simulink model "Encoder_reader_simulink"  (R2025b)
settings: Solver=FixedStepAuto  StartTime=0.0  StopTime=inf  FixedStep=0.01  RelTol=1e-3  EnableMultiTasking=on
libraries: stm32g4xxblockslib x4, stm32f4xxblockslib x2
settings Model: STM32="{\"EncoderBlockForG4\":[{\"ID\":\"untitled:1\"},{\"ID\":\"Lab3_Encoder:1\"},{\"ID\":\"Encoder_reader_simulink:1\"},{\"ID\":\"Encoder_reader_simulink:52\"},{\"ID\":\"Encoder_reader_simulink:53\"},{\"ID\":\"Encoder_reader_simulink:109\"}],\"DigitalPortRead\":[{\"ID\":\"Encoder_reader_simulink:40\"},{\"ID\":\"Encoder_reader_simulink:41\"}]}"  SimulationMode=external  Creator=User  LastModifiedBy=gongk
settings OptimizationCC: DefaultParameterBehavior=Inlined  EnhancedBackFolding=on  PassReuseOutputArgsAs=Individual arguments  ZeroExternalMemoryAtStartup=off  ZeroInternalMemoryAtStartup=off  MaxStackSize=512  OptimizeBlockOrder=speed  DifferentSizesBufferReuse=on  OptimizationCustomize=off  EfficientTunableParamExpr=on
settings DebuggingCC: ParameterTunabilityLossMsg=error
settings HardwareCC: ProdBitPerPointer=32.0  ProdBitPerSizeT=32.0  ProdBitPerPtrDiffT=32.0  ProdLargestAtomicInteger=Long  ProdLargestAtomicFloat=Double  ProdWordSize=32.0  ProdLongLongMode=on  ProdHWDeviceType=ARM Compatible->ARM Cortex-M
settings SFSimCC: MATLABDynamicMemAlloc=off
settings RTWCC: SystemTargetFile=ert.tlc  HardwareBoard=STM32G4xx Based  TemplateMakefile=ert_default_tmf  Toolchain=GNU Tools for ARM Embedded Processors  Description=Embedded Coder
settings CodeAppCC: ForceParamTrailComments=on  IgnoreCustomStorageClasses=off  OperatorAnnotations=on  SimulinkDataObjDesc=on  SFDataObjDesc=on  InsertBlockDesc=on
settings ERTTargetCC: ExtModeTransport=3.0  ExtModeStaticAlloc=on  ExtModeStaticAllocSize=2048.0  ExtModeMexFile=ext_xcp  ExtModeIntrfLevel=Level2 - Open  TargetLangStandard=C99 (ISO)  CodeReplacementLibrary=ARM Cortex-M  SupportContinuousTime=on

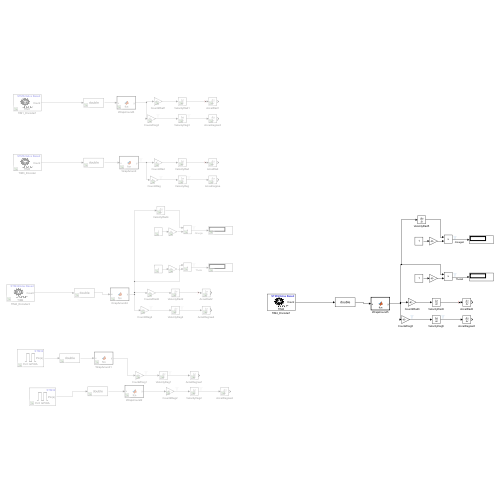
[thumbnail: Simulink's stored preview of the top-level diagram]
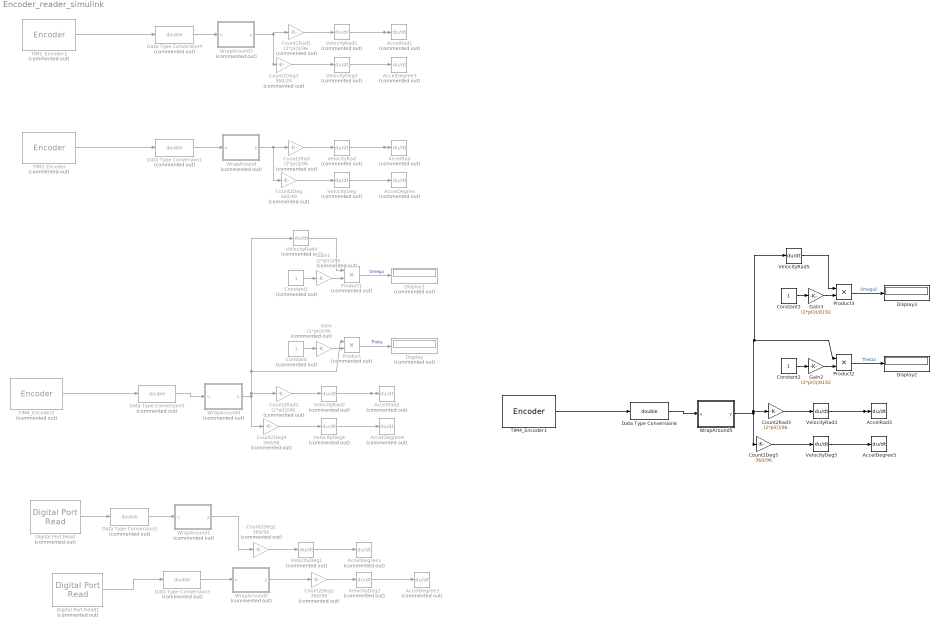
== system Encoder_reader_simulink ==
  AccelDegree{,1..4} (5 alike) : Derivative  Commented=on
  AccelDegree5 : Derivative
  AccelRad : Derivative  Commented=on
  AccelRad1 : Derivative  Commented=on
  AccelRad2 : Derivative  Commented=on
  AccelRad3 : Derivative
  Constant : Constant  Commented=on
  Constant1 : Constant  Commented=on
  Constant2 : Constant
  Constant3 : Constant
  Count2Deg : Gain  Commented=on  Gain=360/48
  Count2Deg1 : Gain  Commented=on  Gain=360/96
  Count2Deg2 : Gain  Commented=on  Gain=360/96
  Count2Deg3 : Gain  Commented=on  Gain=360/24
  Count2Deg4 : Gain  Commented=on  Gain=360/96
  Count2Deg5 : Gain  Gain=360/96
  Count2Rad : Gain  Commented=on  Gain=(2*pi())/96
  Count2Rad1 : Gain  Commented=on  Gain=(2*pi())/96
  Count2Rad2 : Gain  Commented=on  Gain=(2*pi())/96
  Count2Rad3 : Gain  Gain=(2*pi())/96
  Data Type Conversion{1..5} (5 alike) : DataTypeConversion  Commented=on  OutDataTypeStr=double  SaturateOnIntegerOverflow=off  RndMeth=Floor
  Data Type Conversion6 : DataTypeConversion  OutDataTypeStr=double  SaturateOnIntegerOverflow=off  RndMeth=Floor
  Digital Port Read : stm32f4xxblockslib/Digital Port Read  Commented=on  PortName=GPIOA  PinNumber=[4]  ReadOperation=on  IOAsArray=on  SampleTime=-1  EnableSimPort=off  hoistedMaskSrc=ECSoC/ECSimCodegen/Digital Port Read
  Digital Port Read1 : stm32f4xxblockslib/Digital Port Read  Commented=on  PortName=GPIOA  PinNumber=[6]  ReadOperation=on  IOAsArray=on  SampleTime=-1  EnableSimPort=off  hoistedMaskSrc=ECSoC/ECSimCodegen/Digital Port Read
  Display : Display  Commented=on
  Display1 : Display  Commented=on
  Display2 : Display
  Display3 : Display
  Gain : Gain  Commented=on  Gain=(2*pi())/96
  Gain1 : Gain  Commented=on  Gain=(2*pi())/96
  Gain2 : Gain  Gain=(2*pi())/8192
  Gain3 : Gain  Gain=(2*pi())/8192
  Product : Product  Commented=on
  Product1 : Product  Commented=on
  Product2 : Product
  Product3 : Product
  TIM1_Encoder1 : stm32g4xxblockslib/Encoder  Commented=on  TimerModule=TIM1  EnableResetInput=off  OutputCountAfterFirstIndex=off  OutputValidIndex=off  OutputDirection=off  OutputStatus=off  SampleTime=-1
  TIM3_Encoder : stm32g4xxblockslib/Encoder  Commented=on  TimerModule=TIM3  EnableResetInput=off  OutputCountAfterFirstIndex=off  OutputValidIndex=off  OutputDirection=off  OutputStatus=off  SampleTime=-1
  TIM4_Encoder1 : stm32g4xxblockslib/Encoder  TimerModule=TIM4  EnableResetInput=off  OutputCountAfterFirstIndex=off  OutputValidIndex=off  OutputDirection=off  OutputStatus=off  SampleTime=-1
  TIM4_Encoder2 : stm32g4xxblockslib/Encoder  Commented=on  TimerModule=TIM4  EnableResetInput=off  OutputCountAfterFirstIndex=off  OutputValidIndex=off  OutputDirection=off  OutputStatus=off  SampleTime=-1
  VelocityDeg{,1..4} (5 alike) : Derivative  Commented=on
  VelocityDeg5 : Derivative
  VelocityRad{,1..2,4} (4 alike) : Derivative  Commented=on
  VelocityRad3 : Derivative
  VelocityRad5 : Derivative
  WrapAround : MATLAB Function  Commented=on  TreatAsAtomicUnit=on
  WrapAround1 : MATLAB Function  Commented=on  TreatAsAtomicUnit=on
  WrapAround2 : MATLAB Function  Commented=on  TreatAsAtomicUnit=on
  WrapAround3 : MATLAB Function  Commented=on  TreatAsAtomicUnit=on
  WrapAround4 : MATLAB Function  Commented=on  TreatAsAtomicUnit=on
  WrapAround5 : MATLAB Function  TreatAsAtomicUnit=on
  wires:
  TIM3_Encoder/1 -> Data Type Conversion1/1
  Data Type Conversion1/1 -> WrapAround/1(u)
  WrapAround/1(y) -> Count2Deg/1, Count2Rad/1
  Count2Rad/1 -> VelocityRad/1
  Count2Deg/1 -> VelocityDeg/1
  VelocityDeg/1 -> AccelDegree/1
  VelocityRad/1 -> AccelRad/1
  VelocityDeg1/1 -> AccelDegree1/1
  Count2Deg1/1 -> VelocityDeg1/1
  WrapAround1/1(y) -> Count2Deg1/1
  Digital Port Read/1 -> Data Type Conversion2/1
  Data Type Conversion2/1 -> WrapAround1/1(u)
  Digital Port Read1/1 -> Data Type Conversion3/1
  Data Type Conversion3/1 -> WrapAround2/1(u)
  WrapAround2/1(y) -> Count2Deg2/1
  VelocityDeg2/1 -> AccelDegree2/1
  Count2Deg2/1 -> VelocityDeg2/1
  VelocityDeg3/1 -> AccelDegree3/1
  VelocityRad1/1 -> AccelRad1/1
  Count2Deg3/1 -> VelocityDeg3/1
  WrapAround3/1(y) -> Count2Rad1/1, Count2Deg3/1
  Count2Rad1/1 -> VelocityRad1/1
  Data Type Conversion4/1 -> WrapAround3/1(u)
  VelocityDeg4/1 -> AccelDegree4/1
  VelocityRad2/1 -> AccelRad2/1
  Count2Deg4/1 -> VelocityDeg4/1
  WrapAround4/1(y) -> VelocityRad4/1, Product/1, Count2Rad2/1, Count2Deg4/1
  Count2Rad2/1 -> VelocityRad2/1
  Data Type Conversion5/1 -> WrapAround4/1(u)
  TIM4_Encoder2/1 -> Data Type Conversion5/1
  TIM1_Encoder1/1 -> Data Type Conversion4/1
  Constant/1 -> Gain/1
  Gain/1 -> Product/2
  Product/1 -> Display/1  "Theta"
  VelocityRad4/1 -> Product1/1
  Gain1/1 -> Product1/2
  Product1/1 -> Display1/1  "Omega"
  Constant1/1 -> Gain1/1
  Constant3/1 -> Gain3/1
  Gain3/1 -> Product3/2
  Product3/1 -> Display3/1  "Omega2"
  VelocityRad5/1 -> Product3/1
  Gain2/1 -> Product2/2
  Product2/1 -> Display2/1  "Theta2"
  Constant2/1 -> Gain2/1
  Count2Rad3/1 -> VelocityRad3/1
  VelocityDeg5/1 -> AccelDegree5/1
  Count2Deg5/1 -> VelocityDeg5/1
  Data Type Conversion6/1 -> WrapAround5/1(u)
  TIM4_Encoder1/1 -> Data Type Conversion6/1
  VelocityRad3/1 -> AccelRad3/1
  WrapAround5/1(y) -> VelocityRad5/1, Product2/1, Count2Rad3/1, Count2Deg5/1

== matlab function Encoder_reader_simulink/WrapAround ==
  data: u input; y output
function y = fcn(u)
% fcn(u) - ฟังก์ชันสำหรับจัดการ Encoder Wrap-Around
% u: คือ Input (ค่าดิบจาก TIM3 ที่เป็น double)
% y: คือ Output (ค่าตำแหน่งสะสมที่ต่อเนื่อง)

%#codegen

% --- 1. กำหนดค่าคงที่ ---
% ค่า Counter Period (ARR) ที่ตั้งใน IOC คือ 61439
% ดังนั้น จำนวนนับทั้งหมด (States) คือ 61439 + 1 = 61440
persistent PERIOD;
persistent HALF_PERIOD;

% --- 2. สร้างตัวแปร "จำ" ค่า (Persistent Variables) ---
% persistent คือตัวแปรที่ "จำ" ค่าของตัวเองไว้ได้ แม้ฟังก์ชันจะรันจบไปแล้ว
persistent last_raw_count;    % เก็บค่าดิบจาก TIM3 ครั้งล่าสุด
persistent accumulated_count; % เก็บค่าตำแหน่งสะสม (Output)

% --- 3. การรันครั้งแรก (Initialization) ---
% isempty() จะเป็นจริงแค่ครั้งแรกที่ Simulink เริ่มรัน
if isempty(PERIOD)
    PERIOD        = 61440.0; % 61439 + 1 (ใช้ .0 เพื่อให้เป็น double)
    HALF_PERIOD   = PERIOD / 2.0; % 30720.0 
end

if isempty(last_raw_count)
    % ถ้าเป็นครั้งแรก ให้ตั้งค่าเริ่มต้น
    last_raw_count    = u;
    accumulated_count = 0.0;
else
    % --- 4. การรันครั้งถัดๆ ไป (คำนวณหาค่าต่าง) ---
    
    % หาผลต่างดิบ (Raw Delta)
    delta = u - last_raw_count;
    
    % --- 5. ตรวจจับการวนกลับ (Wrap-Around Detection) ---
    
    if delta < -HALF_PERIOD
        % เกิด Overflow (เช่น จาก 61439 -> 0, delta จะประมาณ -61439)
        % นี่คือการหมุนไปข้างหน้า (+1)
        delta = delta + PERIOD; % แก้ไข: -61439 + 61440 = +1
        
    elseif delta > HALF_PERIOD
        % เกิด Underflow (เช่น จาก 0 -> 61439, delta จะประมาณ +61439)
        % นี่คือการหมุนย้อนกลับ (-1)
        delta = delta - PERIOD; % แก้ไข: +61439 - 61440 = -1
    
    % else: (ถ้า delta อยู่ในช่วง +/- 30720)
        % ไม่มีการวนกลับ, 'delta' ถูกต้องแล้ว
    end
    
    % --- 6. อัปเดตค่าสะสม และค่าล่าสุด ---
    
    % บวกค่า delta ที่แก้ไขแล้ว เข้าไปในค่าสะสม
    accumulated_count = accumulated_count + delta;


    
    % "จำ" ค่าดิบครั้งนี้ไว้ เพื่อใช้ในรอบถัดไป
    last_raw_count = u;
end

% --- 7. ส่งค่า Output ---
y = accumulated_count;

end

== matlab function Encoder_reader_simulink/WrapAround2 ==
  data: u input; y output
function y = fcn(u)
% fcn(u) - ฟังก์ชันสำหรับจัดการ Encoder Wrap-Around
% u: คือ Input (ค่าดิบจาก TIM3 ที่เป็น double)
% y: คือ Output (ค่าตำแหน่งสะสมที่ต่อเนื่อง)

%#codegen

% --- 1. กำหนดค่าคงที่ ---
% ค่า Counter Period (ARR) ที่ตั้งใน IOC คือ 61439
% ดังนั้น จำนวนนับทั้งหมด (States) คือ 61439 + 1 = 61440
persistent PERIOD;
persistent HALF_PERIOD;

% --- 2. สร้างตัวแปร "จำ" ค่า (Persistent Variables) ---
% persistent คือตัวแปรที่ "จำ" ค่าของตัวเองไว้ได้ แม้ฟังก์ชันจะรันจบไปแล้ว
persistent last_raw_count;    % เก็บค่าดิบจาก TIM3 ครั้งล่าสุด
persistent accumulated_count; % เก็บค่าตำแหน่งสะสม (Output)

% --- 3. การรันครั้งแรก (Initialization) ---
% isempty() จะเป็นจริงแค่ครั้งแรกที่ Simulink เริ่มรัน
if isempty(PERIOD)
    PERIOD        = 1024.0; % 61439 + 1 (ใช้ .0 เพื่อให้เป็น double)
    HALF_PERIOD   = PERIOD / 2.0; % 30720.0 
end

if isempty(last_raw_count)
    % ถ้าเป็นครั้งแรก ให้ตั้งค่าเริ่มต้น
    last_raw_count    = u;
    accumulated_count = u;
else
    % --- 4. การรันครั้งถัดๆ ไป (คำนวณหาค่าต่าง) ---
    
    % หาผลต่างดิบ (Raw Delta)
    delta = u - last_raw_count;
    
    % --- 5. ตรวจจับการวนกลับ (Wrap-Around Detection) ---
    
    if delta < -HALF_PERIOD
        % เกิด Overflow (เช่น จาก 61439 -> 0, delta จะประมาณ -61439)
        % นี่คือการหมุนไปข้างหน้า (+1)
        delta = delta + PERIOD; % แก้ไข: -61439 + 61440 = +1
        
    elseif delta > HALF_PERIOD
        % เกิด Underflow (เช่น จาก 0 -> 61439, delta จะประมาณ +61439)
        % นี่คือการหมุนย้อนกลับ (-1)
        delta = delta - PERIOD; % แก้ไข: +61439 - 61440 = -1
    
    % else: (ถ้า delta อยู่ในช่วง +/- 30720)
        % ไม่มีการวนกลับ, 'delta' ถูกต้องแล้ว
    end
    
    % --- 6. อัปเดตค่าสะสม และค่าล่าสุด ---
    
    % บวกค่า delta ที่แก้ไขแล้ว เข้าไปในค่าสะสม
    accumulated_count = accumulated_count + delta;
    
    % "จำ" ค่าดิบครั้งนี้ไว้ เพื่อใช้ในรอบถัดไป
    last_raw_count = u;
end

% --- 7. ส่งค่า Output ---
y = accumulated_count;

end

== matlab function Encoder_reader_simulink/WrapAround3 ==
  data: u input; y output
function y = fcn(u)
% fcn(u) - ฟังก์ชันสำหรับจัดการ Encoder Wrap-Around
% u: คือ Input (ค่าดิบจาก TIM3 ที่เป็น double)
% y: คือ Output (ค่าตำแหน่งสะสมที่ต่อเนื่อง)

%#codegen

% --- 1. กำหนดค่าคงที่ ---
% ค่า Counter Period (ARR) ที่ตั้งใน IOC คือ 61439
% ดังนั้น จำนวนนับทั้งหมด (States) คือ 61439 + 1 = 61440
persistent PERIOD;
persistent HALF_PERIOD;

% --- 2. สร้างตัวแปร "จำ" ค่า (Persistent Variables) ---
% persistent คือตัวแปรที่ "จำ" ค่าของตัวเองไว้ได้ แม้ฟังก์ชันจะรันจบไปแล้ว
persistent last_raw_count;    % เก็บค่าดิบจาก TIM3 ครั้งล่าสุด
persistent accumulated_count; % เก็บค่าตำแหน่งสะสม (Output)

% --- 3. การรันครั้งแรก (Initialization) ---
% isempty() จะเป็นจริงแค่ครั้งแรกที่ Simulink เริ่มรัน
if isempty(PERIOD)
    PERIOD        = 61440.0; % 61439 + 1 (ใช้ .0 เพื่อให้เป็น double)
    HALF_PERIOD   = PERIOD / 2.0; % 30720.0 
end

if isempty(last_raw_count)
    % ถ้าเป็นครั้งแรก ให้ตั้งค่าเริ่มต้น
    last_raw_count    = u;
    accumulated_count = 0.0;
else
    % --- 4. การรันครั้งถัดๆ ไป (คำนวณหาค่าต่าง) ---
    
    % หาผลต่างดิบ (Raw Delta)
    delta = u - last_raw_count;
    
    % --- 5. ตรวจจับการวนกลับ (Wrap-Around Detection) ---
    
    if delta < -HALF_PERIOD
        % เกิด Overflow (เช่น จาก 61439 -> 0, delta จะประมาณ -61439)
        % นี่คือการหมุนไปข้างหน้า (+1)
        delta = delta + PERIOD; % แก้ไข: -61439 + 61440 = +1
        
    elseif delta > HALF_PERIOD
        % เกิด Underflow (เช่น จาก 0 -> 61439, delta จะประมาณ +61439)
        % นี่คือการหมุนย้อนกลับ (-1)
        delta = delta - PERIOD; % แก้ไข: +61439 - 61440 = -1
    
    % else: (ถ้า delta อยู่ในช่วง +/- 30720)
        % ไม่มีการวนกลับ, 'delta' ถูกต้องแล้ว
    end
    
    % --- 6. อัปเดตค่าสะสม และค่าล่าสุด ---
    
    % บวกค่า delta ที่แก้ไขแล้ว เข้าไปในค่าสะสม
    accumulated_count = accumulated_count + delta;

    
    % "จำ" ค่าดิบครั้งนี้ไว้ เพื่อใช้ในรอบถัดไป
    last_raw_count = u;
end

% --- 7. ส่งค่า Output ---
y = accumulated_count;

end

== matlab function Encoder_reader_simulink/WrapAround4 ==
  data: u input; y output
function y = fcn(u)
% fcn(u) - ฟังก์ชันสำหรับจัดการ Encoder Wrap-Around
% u: คือ Input (ค่าดิบจาก TIM3 ที่เป็น double)
% y: คือ Output (ค่าตำแหน่งสะสมที่ต่อเนื่อง)

%#codegen

% --- 1. กำหนดค่าคงที่ ---
% ค่า Counter Period (ARR) ที่ตั้งใน IOC คือ 61439
% ดังนั้น จำนวนนับทั้งหมด (States) คือ 61439 + 1 = 61440
persistent PERIOD;
persistent HALF_PERIOD;

% --- 2. สร้างตัวแปร "จำ" ค่า (Persistent Variables) ---
% persistent คือตัวแปรที่ "จำ" ค่าของตัวเองไว้ได้ แม้ฟังก์ชันจะรันจบไปแล้ว
persistent last_raw_count;    % เก็บค่าดิบจาก TIM3 ครั้งล่าสุด
persistent accumulated_count; % เก็บค่าตำแหน่งสะสม (Output)

% --- 3. การรันครั้งแรก (Initialization) ---
% isempty() จะเป็นจริงแค่ครั้งแรกที่ Simulink เริ่มรัน
if isempty(PERIOD)
    PERIOD        = 61440.0; % 61439 + 1 (ใช้ .0 เพื่อให้เป็น double)
    HALF_PERIOD   = PERIOD / 2.0; % 30720.0 
end

if isempty(last_raw_count)
    % ถ้าเป็นครั้งแรก ให้ตั้งค่าเริ่มต้น
    last_raw_count    = u;
    accumulated_count = 0.0;
else
    % --- 4. การรันครั้งถัดๆ ไป (คำนวณหาค่าต่าง) ---
    
    % หาผลต่างดิบ (Raw Delta)
    delta = u - last_raw_count;
    
    % --- 5. ตรวจจับการวนกลับ (Wrap-Around Detection) ---
    
    if delta < -HALF_PERIOD
        % เกิด Overflow (เช่น จาก 61439 -> 0, delta จะประมาณ -61439)
        % นี่คือการหมุนไปข้างหน้า (+1)
        delta = delta + PERIOD; % แก้ไข: -61439 + 61440 = +1
        
    elseif delta > HALF_PERIOD
        % เกิด Underflow (เช่น จาก 0 -> 61439, delta จะประมาณ +61439)
        % นี่คือการหมุนย้อนกลับ (-1)
        delta = delta - PERIOD; % แก้ไข: +61439 - 61440 = -1
    
    % else: (ถ้า delta อยู่ในช่วง +/- 30720)
        % ไม่มีการวนกลับ, 'delta' ถูกต้องแล้ว
    end
    
    % --- 6. อัปเดตค่าสะสม และค่าล่าสุด ---
    
    % บวกค่า delta ที่แก้ไขแล้ว เข้าไปในค่าสะสม
    accumulated_count = accumulated_count + delta;


    
    % "จำ" ค่าดิบครั้งนี้ไว้ เพื่อใช้ในรอบถัดไป
    last_raw_count = u;
end

% --- 7. ส่งค่า Output ---
y = accumulated_count;

end

== matlab function Encoder_reader_simulink/WrapAround5 ==
  data: u input; y output
function y = fcn(u)
% fcn(u) - ฟังก์ชันสำหรับจัดการ Encoder Wrap-Around
% u: คือ Input (ค่าดิบจาก TIM3 ที่เป็น double)
% y: คือ Output (ค่าตำแหน่งสะสมที่ต่อเนื่อง)

%#codegen

% --- 1. กำหนดค่าคงที่ ---
% ค่า Counter Period (ARR) ที่ตั้งใน IOC คือ 61439
% ดังนั้น จำนวนนับทั้งหมด (States) คือ 61439 + 1 = 61440
persistent PERIOD;
persistent HALF_PERIOD;

% --- 2. สร้างตัวแปร "จำ" ค่า (Persistent Variables) ---
% persistent คือตัวแปรที่ "จำ" ค่าของตัวเองไว้ได้ แม้ฟังก์ชันจะรันจบไปแล้ว
persistent last_raw_count;    % เก็บค่าดิบจาก TIM3 ครั้งล่าสุด
persistent accumulated_count; % เก็บค่าตำแหน่งสะสม (Output)

% --- 3. การรันครั้งแรก (Initialization) ---
% isempty() จะเป็นจริงแค่ครั้งแรกที่ Simulink เริ่มรัน
if isempty(PERIOD)
    PERIOD        = 61440.0; % 61439 + 1 (ใช้ .0 เพื่อให้เป็น double)
    HALF_PERIOD   = PERIOD / 2.0; % 30720.0 
end

if isempty(last_raw_count)
    % ถ้าเป็นครั้งแรก ให้ตั้งค่าเริ่มต้น
    last_raw_count    = u;
    accumulated_count = 0.0;
else
    % --- 4. การรันครั้งถัดๆ ไป (คำนวณหาค่าต่าง) ---
    
    % หาผลต่างดิบ (Raw Delta)
    delta = u - last_raw_count;
    
    % --- 5. ตรวจจับการวนกลับ (Wrap-Around Detection) ---
    
    if delta < -HALF_PERIOD
        % เกิด Overflow (เช่น จาก 61439 -> 0, delta จะประมาณ -61439)
        % นี่คือการหมุนไปข้างหน้า (+1)
        delta = delta + PERIOD; % แก้ไข: -61439 + 61440 = +1
        
    elseif delta > HALF_PERIOD
        % เกิด Underflow (เช่น จาก 0 -> 61439, delta จะประมาณ +61439)
        % นี่คือการหมุนย้อนกลับ (-1)
        delta = delta - PERIOD; % แก้ไข: +61439 - 61440 = -1
    
    % else: (ถ้า delta อยู่ในช่วง +/- 30720)
        % ไม่มีการวนกลับ, 'delta' ถูกต้องแล้ว
    end
    
    % --- 6. อัปเดตค่าสะสม และค่าล่าสุด ---
    
    % บวกค่า delta ที่แก้ไขแล้ว เข้าไปในค่าสะสม
    accumulated_count = accumulated_count + delta;


    
    % "จำ" ค่าดิบครั้งนี้ไว้ เพื่อใช้ในรอบถัดไป
    last_raw_count = u;
end

% --- 7. ส่งค่า Output ---
y = accumulated_count;

end

== matlab function Encoder_reader_simulink/WrapAround1 ==
  data: u input; y output
function y = fcn(u)
% fcn(u) - ฟังก์ชันสำหรับจัดการ Encoder Wrap-Around
% u: คือ Input (ค่าดิบจาก TIM3 ที่เป็น double)
% y: คือ Output (ค่าตำแหน่งสะสมที่ต่อเนื่อง)

%#codegen

% --- 1. กำหนดค่าคงที่ ---
% ค่า Counter Period (ARR) ที่ตั้งใน IOC คือ 61439
% ดังนั้น จำนวนนับทั้งหมด (States) คือ 61439 + 1 = 61440
persistent PERIOD;
persistent HALF_PERIOD;

% --- 2. สร้างตัวแปร "จำ" ค่า (Persistent Variables) ---
% persistent คือตัวแปรที่ "จำ" ค่าของตัวเองไว้ได้ แม้ฟังก์ชันจะรันจบไปแล้ว
persistent last_raw_count;    % เก็บค่าดิบจาก TIM3 ครั้งล่าสุด
persistent accumulated_count; % เก็บค่าตำแหน่งสะสม (Output)

% --- 3. การรันครั้งแรก (Initialization) ---
% isempty() จะเป็นจริงแค่ครั้งแรกที่ Simulink เริ่มรัน
if isempty(PERIOD)
    PERIOD        = 1024.0; % 61439 + 1 (ใช้ .0 เพื่อให้เป็น double)
    HALF_PERIOD   = PERIOD / 2.0; % 30720.0 
end

if isempty(last_raw_count)
    % ถ้าเป็นครั้งแรก ให้ตั้งค่าเริ่มต้น
    last_raw_count    = u;
    accumulated_count = u;
else
    % --- 4. การรันครั้งถัดๆ ไป (คำนวณหาค่าต่าง) ---
    
    % หาผลต่างดิบ (Raw Delta)
    delta = u - last_raw_count;
    
    % --- 5. ตรวจจับการวนกลับ (Wrap-Around Detection) ---
    
    if delta < -HALF_PERIOD
        % เกิด Overflow (เช่น จาก 61439 -> 0, delta จะประมาณ -61439)
        % นี่คือการหมุนไปข้างหน้า (+1)
        delta = delta + PERIOD; % แก้ไข: -61439 + 61440 = +1
        
    elseif delta > HALF_PERIOD
        % เกิด Underflow (เช่น จาก 0 -> 61439, delta จะประมาณ +61439)
        % นี่คือการหมุนย้อนกลับ (-1)
        delta = delta - PERIOD; % แก้ไข: +61439 - 61440 = -1
    
    % else: (ถ้า delta อยู่ในช่วง +/- 30720)
        % ไม่มีการวนกลับ, 'delta' ถูกต้องแล้ว
    end
    
    % --- 6. อัปเดตค่าสะสม และค่าล่าสุด ---
    
    % บวกค่า delta ที่แก้ไขแล้ว เข้าไปในค่าสะสม
    accumulated_count = accumulated_count + delta;
    
    % "จำ" ค่าดิบครั้งนี้ไว้ เพื่อใช้ในรอบถัดไป
    last_raw_count = u;
end

% --- 7. ส่งค่า Output ---
y = accumulated_count;

end
